simulink model "SystemPartModel"  (Simulink 8.8)
settings: Solver=VariableStepAuto  StartTime=0.0  StopTime=24*6  RelTol=1e-3
libraries: mpclib x1
settings Model: Creator=zhu  LastModifiedBy=山楂
settings SolverCC: ZeroCrossAlgorithm=Adaptive
settings DataIOCC: LimitDataPoints=off  SaveFormat=Dataset  SignalLoggingSaveFormat=Dataset  ReturnWorkspaceOutputs=on
settings OptimizationCC: LifeSpan=auto
settings DebuggingCC: UnderspecifiedInitializationDetection=Simplified  MergeDetectMultiDrivingBlocksExec=error  IgnoredZcDiagnostic=none  FcnCallInpInsideContextMsg=error  StateNameClashWarn=none  SFUnexpectedBacktrackingDiag=error  SFNoUnconditionalDefaultTransitionDiag=error  SFExecutionAtInitializationDiag=warning
settings HardwareCC: ProdBitPerPointer=64  ProdBitPerSizeT=64  ProdBitPerPtrDiffT=64  ProdLargestAtomicFloat=Float  ProdIntDivRoundTo=Zero  ProdEndianess=LittleEndian  ProdWordSize=64  ProdHWDeviceType=Intel->x86-64 (Windows64)
settings ModelReferenceCC: PropagateSignalLabelsOutOfModel=on
settings SFSimCC: SimUseLocalCustomCode=on
settings RTWCC: RTWUseLocalCustomCode=on
settings GRTTargetCC: TargetLangStandard=C99 (ISO)  CombineOutputUpdateFcns=on  GRTInterface=off
settings ConfigComp: CovMetricSettings=dwe  CovSaveCumulativeToWorkspaceVar=off  CovSaveSingleToWorkspaceVar=off  CovExternalEMLEnable=on

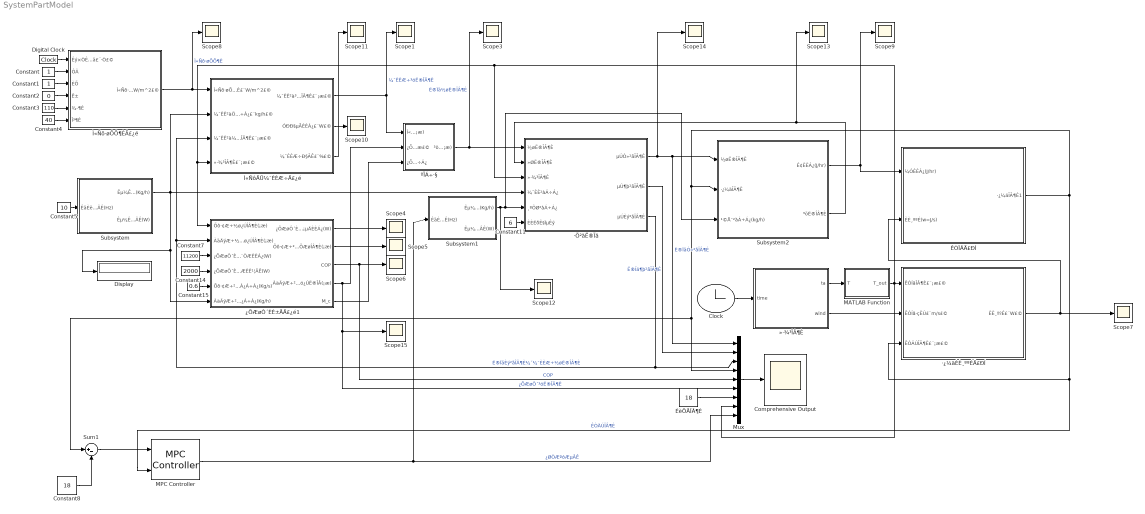
== system SystemPartModel ==
  Clock : Clock
      mask Display: image('$imagefile'); % Use "Edit Image" on toolstrip to change.
  Comprehensive Output : Scope
  Constant : Constant
  Constant1 : Constant
  Constant11 : Constant  Value=6
  Constant14 : Constant  Value=2000
  Constant15 : Constant  Value=0.6
  Constant2 : Constant  Value=0
  Constant3 : Constant  Value=110
  Constant4 : Constant  Value=40
  Constant5 : Constant  Value=10
  Constant7 : Constant  Value=11200
  Constant8 : Constant  Value=18
  Digital Clock : DigitalClock
  Display : Display
  MATLAB Function : MATLAB Function  TreatAsAtomicUnit=on
  MPC Controller : mpclib/MPC Controller  SCDEnableBlockLinearizationSpecification=on  is_multiple=0  enable_value=0  return_u0=off  updateMPCinCallerWorkspace=on  md_inport=off  mv_inport=off  uref_inport=off  cost_outport=off  return_sequence=off  return_qpstatus=off  return_xseq=off  return_state=off  return_ovseq=off  state_inport=off  umin_inport=off  umax_inport=off  ymin_inport=off  ymax_inport=off  cc_inport=off  ywt_inport=off  uwt_inport=off  duwt_inport=off  rhoeps_inport=off  pm_inport=off  MaximumP=10  HorizonChoice=FixedHorizon  n_ts=1  n_p=10  n_mv=1  n_md=1  n_ud=0  n_mo=1  n_uo=0  BlockDataType=double  SampleTimeInherited=off  switch_inport=off
  Mux : Mux  Inputs=9
  Scope{1,3..15} (14 alike) : Scope
  Subsystem : Subsystem
      mask Display: image('$imagefile'); % Use "Edit Image" on toolstrip to change.
  Subsystem1 : Subsystem
      mask Display: image('$imagefile'); % Use "Edit Image" on toolstrip to change.
  Subsystem2 : Subsystem
  Sum1 : Sum  Inputs=|+-
  分层水箱 : Subsystem
      mask Display: image('$imagefile'); % Use "Edit Image" on toolstrip to change.
  合流阀 : Subsystem
      mask Display: image('$imagefile'); % Use "Edit Image" on toolstrip to change.
  太阳能集热器模块 : Subsystem  mask{cw=4187, Ac=40, Mc=1000, UL=1, tau_alpha=0.86}
      mask prompts: cw "水定压比热容，J/kg*℃"; Ac "集热面积，m^2"; Mc "集热器贮水质量，kg"; UL "集热器热损系数，W/m^2"; tau_alpha "透射比和吸收比乘积有效系数"
      mask DialogControl DescGroupVar Prompt: 太阳能集热器模块
      mask Display: image('$imagefile'); % Use "Edit Image" on toolstrip to change.
  太阳辐照度模块 : Subsystem
      mask Display: image('$imagefile'); % Use "Edit Image" on toolstrip to change.
  室温模型 : Subsystem  mask{rou=1.29, ca=1003, V=423}
      mask prompts: rou "空气密度,kg/m^3"; ca "比热容,J/kg*K"; V "室内容积，m^3"
      mask Display: image('$imagefile'); % Use "Edit Image" on toolstrip to change.
  房间热负荷模型 : Subsystem
      mask Display: image('$imagefile'); % Use "Edit Image" on toolstrip to change.
  环境温度 : MATLAB Function  TreatAsAtomicUnit=on
  空气源热泵模块1 : Subsystem
      mask Display: image('$imagefile'); % Use "Edit Image" on toolstrip to change.
  设置温度 : Constant  Value=18
  wires:
  Digital Clock/1 -> 太阳辐照度模块/1(数字时间（分）)
  Constant/1 -> 太阳辐照度模块/2(月)
  Constant1/1 -> 太阳辐照度模块/3(日)
  Constant2/1 -> 太阳辐照度模块/4(时)
  Constant3/1 -> 太阳辐照度模块/5(经度)
  Constant4/1 -> 太阳辐照度模块/6(纬度)
  太阳辐照度模块/1(太阳辐照度（W/m^2）) -> Scope8/1, 太阳能集热器模块/1(太阳辐照度（W/m^2）)  "太阳辐照度"
  合流阀/1(出水温度(℃)) -> 分层水箱/1(进水温度), Scope3/1  "水箱进水温度"
  空气源热泵模块1/5(M_c) -> 合流阀/3(空气源流量)
  空气源热泵模块1/4(冷凝器侧出口水温(℃)) -> Mux/6, Scope15/1, 合流阀/2(空气源侧来水温度(℃）)  "空气源出水温度"
  太阳能集热器模块/1(集热侧出水温度（℃）) -> Scope1/1, 合流阀/1(太阳能侧来水温度(℃))  "集热器出水温度"
  分层水箱/1(第一层温度) -> Scope14/1, Subsystem2/1(进水温度), Mux/1  "水箱一层温度"
  Subsystem2/2(出水温度) -> Scope13/1, 分层水箱/2(回水温度)
  Constant11/1 -> 分层水箱/6(热损失系数)
  Constant7/1 -> 空气源热泵模块1/3(空气源热泵额定制热量(W))
  Constant14/1 -> 空气源热泵模块1/4(空气源热泵额定制热功率(W))
  Constant15/1 -> 空气源热泵模块1/5(蒸发器侧介质的质量流量(Kg/s))
  Mux/1 -> Comprehensive Output/1
  分层水箱/2(第二层温度) -> Mux/2  "水箱二层温度"
  分层水箱/3(第三层温度) -> 空气源热泵模块1/2(冷凝器进口温度(℃)), 太阳能集热器模块/3(集热侧进水温度（℃）), Mux/3  "水箱三层温度即集热器进水温度"
  空气源热泵模块1/1(空气源热泵蒸发器从热源侧提取的热量(W)) -> Scope4/1
  空气源热泵模块1/2(蒸发器侧出口空气温度(℃)) -> Scope5/1
  空气源热泵模块1/3(COP) -> Mux/5, Scope6/1  "COP"
  太阳能集热器模块/2(有效得热量（W）) -> Scope10/1
  太阳能集热器模块/3(集热器效率（%）) -> Scope11/1
  Constant5/1 -> Subsystem/1(输入频率(Hz))
  Subsystem/1(实际输出流量(Kg/h)) -> 太阳能集热器模块/2(集热侧质量流量（kg/h）), 分层水箱/4(集热侧流量), Display/1, 空气源热泵模块1/6(冷凝器侧介质的质量流量(Kg/h))
  环境温度/1(ta) -> MATLAB Function/1(T)
  环境温度/2(wind) -> 房间热负荷模型/2(室外风速（m/s）)
  Clock/1 -> 环境温度/1(time)
  室温模型/1(房间温度1) -> Subsystem2/2(房间温度), Sum1/1, Mux/4, MPC Controller/2, 房间热负荷模型/3(室内温度（℃）)  "室内温度"
  Subsystem1/1(实际输出流量(Kg/h)) -> Scope12/1, Subsystem2/3(供暖侧流量(kg/h)), 分层水箱/5(负载侧流量)
  Subsystem2/1(散热量(J/hr)) -> 室温模型/1(加热量(J/hr)), Scope9/1
  设置温度/1 -> Mux/7
  房间热负荷模型/1(热负荷（W）) -> 室温模型/2(热负荷(w=J/s)), Scope7/1
  MPC Controller/1 -> Mux/9, Subsystem1/1(输入频率(Hz))  "控制后频率"
  Constant8/1 -> Sum1/2
  MATLAB Function/1(T_out) -> Mux/8, 房间热负荷模型/1(室外温度（℃）), 分层水箱/3(环境温度), 空气源热泵模块1/1(蒸发器进口温度(℃)), 太阳能集热器模块/4(环境温度（℃）)
  Sum1/1 -> MPC Controller/1

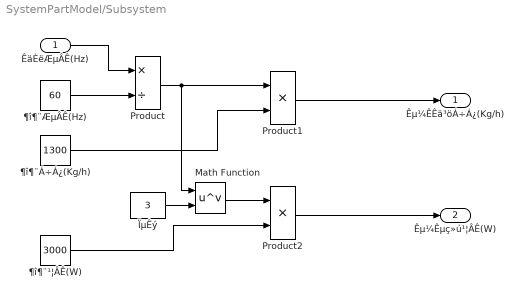
== system SystemPartModel/Subsystem ==
  输入频率(Hz) : Inport
  Math Function : Math  Operator=pow  SaturateOnIntegerOverflow=on
  Product : Product  Inputs=*/
  Product1 : Product
  Product2 : Product
  系数 : Constant  Value=3
  额定功率(W) : Constant  Value=3000
  额定流量(Kg/h) : Constant  Value=1300
  额定频率(Hz) : Constant  Value=60
  实际输出流量(Kg/h) : Outport
  实际电机功率(W) : Outport  Port=2
  wires:
  系数/1 -> Math Function/2
  Math Function/1 -> Product2/1
  额定频率(Hz)/1 -> Product/2
  额定流量(Kg/h)/1 -> Product1/2
  Product/1 -> Math Function/1, Product1/1
  额定功率(W)/1 -> Product2/2
  Product2/1 -> 实际电机功率(W)/1
  输入频率(Hz)/1 -> Product/1
  Product1/1 -> 实际输出流量(Kg/h)/1

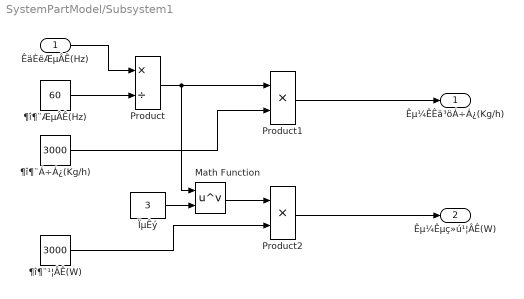
== system SystemPartModel/Subsystem1 ==
  输入频率(Hz) : Inport
  Math Function : Math  Operator=pow  SaturateOnIntegerOverflow=on
  Product : Product  Inputs=*/
  Product1 : Product
  Product2 : Product
  系数 : Constant  Value=3
  额定功率(W) : Constant  Value=3000
  额定流量(Kg/h) : Constant  Value=3000
  额定频率(Hz) : Constant  Value=60
  实际输出流量(Kg/h) : Outport
  实际电机功率(W) : Outport  Port=2
  wires:
  Product1/1 -> 实际输出流量(Kg/h)/1
  输入频率(Hz)/1 -> Product/1
  Product2/1 -> 实际电机功率(W)/1
  额定功率(W)/1 -> Product2/2
  Product/1 -> Product1/1, Math Function/1
  额定流量(Kg/h)/1 -> Product1/2
  额定频率(Hz)/1 -> Product/2
  Math Function/1 -> Product2/1
  系数/1 -> Math Function/2

== system SystemPartModel/Subsystem2 ==
  进水温度 : Inport
  房间温度 : Inport  Port=2
  供暖侧流量(kg/h) : Inport  Port=3
  Constant : Constant  Value=7.77
  Subsystem : Subsystem
  Subsystem1 : Subsystem
  散热量(J/hr) : Outport
  出水温度 : Outport  Port=2
  wires:
  房间温度/1 -> Subsystem/2(房间温度)
  进水温度/1 -> Subsystem1/3(进水温度), Subsystem/1(进水温度)
  Constant/1 -> ?
  Subsystem1/1(出水温度) -> 出水温度/1
  供暖侧流量(kg/h)/1 -> Subsystem1/2(供热流量(kg/h)), Subsystem/3(供热流量，kg/h)
  Subsystem/1(散热量(j/hr)) -> 散热量(J/hr)/1, Subsystem1/1(散热量)

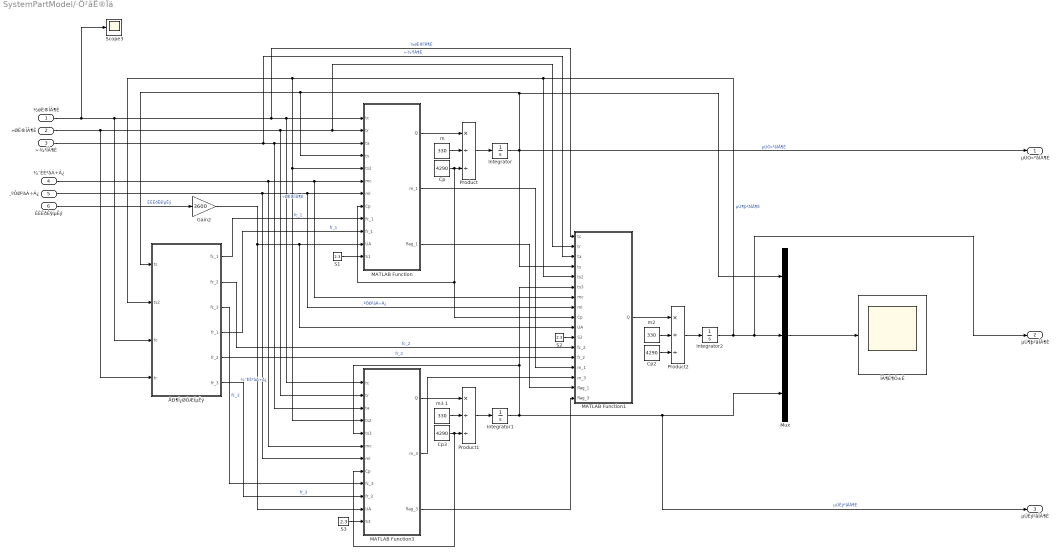
== system SystemPartModel/分层水箱 ==
  进水温度 : Inport
  回水温度 : Inport  Port=2
  环境温度 : Inport  Port=3
  集热侧流量 : Inport  Port=4
  负载侧流量 : Inport  Port=5
  热损失系数 : Inport  Port=6
  Cp : Constant  Value=4290
  Cp2 : Constant  Value=4290
  Cp3 : Constant  Value=4290
  Gain2 : Gain  Gain=3600
  Integrator : Integrator  InitialCondition=45
  Integrator1 : Integrator  InitialCondition=45
  Integrator2 : Integrator  InitialCondition=45
  MATLAB Function : MATLAB Function  TreatAsAtomicUnit=on
  MATLAB Function1 : MATLAB Function  TreatAsAtomicUnit=on
  MATLAB Function3 : MATLAB Function  TreatAsAtomicUnit=on
  Mux : Mux  Inputs=3
  Product : Product  Inputs=*//
  Product1 : Product  Inputs=*//
  Product2 : Product  Inputs=*//
  S1 : Constant  Value=2.3
  S2 : Constant  Value=2.3
  S3 : Constant  Value=2.3
  Scope3 : Scope
  "m " : Constant  Value=330
  m2 : Constant  Value=330
  m3 1 : Constant  Value=330
  判断控制系数 : MATLAB Function  TreatAsAtomicUnit=on
  温度对比 : Scope
  第一层温度 : Outport
  第二层温度 : Outport  Port=2
  第三层温度 : Outport  Port=3
  wires:
  Integrator1/1 -> 第三层温度/1, Mux/3, MATLAB Function1/6(ts3), MATLAB Function3/5(ts3)  "第三层温度"
  Integrator2/1 -> 第二层温度/1, Mux/2, MATLAB Function1/5(ts2), MATLAB Function3/4(ts2), MATLAB Function/5(ts2), 判断控制系数/2(ts2)  "第二层温度"
  Product/1 -> Integrator/1
  负载侧流量/1 -> MATLAB Function3/7(ml), MATLAB Function1/8(ml), MATLAB Function/7(ml)  "负载侧流量"
  Integrator/1 -> 第一层温度/1, MATLAB Function/4(ts), 判断控制系数/1(ts), Mux/1, MATLAB Function1/4(ts)  "第一层温度"
  Mux/1 -> 温度对比/1
  MATLAB Function/3(flag_1) -> MATLAB Function1/16(flag_1)
  "m "/1 -> Product/2
  判断控制系数/5(fr_2) -> MATLAB Function1/13(fr_2)  "fr_2"
  MATLAB Function3/1(Q) -> Product1/1
  判断控制系数/4(fr_1) -> MATLAB Function/10(fr_1)  "fr_1"
  环境温度/1 -> MATLAB Function1/3(ta), MATLAB Function3/3(ta), MATLAB Function/3(ta)  "环境温度"
  判断控制系数/1(fc_1) -> MATLAB Function/9(fc_1)  "fc_1"
  MATLAB Function3/3(flag_3) -> MATLAB Function1/17(flag_3)
  Product1/1 -> Integrator1/1
  判断控制系数/3(fc_3) -> MATLAB Function3/9(fc_3)  "fc_3"
  回水温度/1 -> 判断控制系数/4(tr), MATLAB Function1/2(tr), MATLAB Function/2(tr), MATLAB Function3/2(tr)  "回水温度"
  m3 1/1 -> Product1/2
  MATLAB Function1/1(Q) -> Product2/1
  Cp3/1 -> MATLAB Function3/8(Cp), Product1/3
  MATLAB Function/1(Q) -> Product/1
  判断控制系数/2(fc_2) -> MATLAB Function1/12(fc_2)  "fc_2"
  m2/1 -> Product2/2
  Cp2/1 -> Product2/3
  判断控制系数/6(fr_3) -> MATLAB Function3/10(fr_3)  "fr_3"
  热损失系数/1 -> Gain2/1  "热损失系数"
  Cp/1 -> MATLAB Function1/9(Cp), MATLAB Function/8(Cp), Product/3
  S1/1 -> MATLAB Function/12(S1)
  S3/1 -> MATLAB Function3/12(S3)
  集热侧流量/1 -> MATLAB Function3/6(mc), MATLAB Function1/7(mc), MATLAB Function/6(mc)  "集热侧流量"
  S2/1 -> MATLAB Function1/11(S2)
  MATLAB Function3/2(m_3) -> MATLAB Function1/15(m_3)
  进水温度/1 -> Scope3/1, 判断控制系数/3(tc), MATLAB Function1/1(tc), MATLAB Function3/1(tc), MATLAB Function/1(tc)  "进水温度"
  MATLAB Function/2(m_1) -> MATLAB Function1/14(m_1)
  Product2/1 -> Integrator2/1
  Gain2/1 -> MATLAB Function3/11(UA), MATLAB Function1/10(UA), MATLAB Function/11(UA)

== system SystemPartModel/合流阀 ==
  太阳能侧来水温度(℃) : Inport
  空气源侧来水温度(℃） : Inport  Port=2
  空气源流量 : Inport  Port=3
  MATLAB Function : MATLAB Function  TreatAsAtomicUnit=on
  出水温度(℃) : Outport
  wires:
  太阳能侧来水温度(℃)/1 -> MATLAB Function/1(c_in)
  空气源侧来水温度(℃）/1 -> MATLAB Function/2(a_in)
  MATLAB Function/1(t_out) -> 出水温度(℃)/1
  空气源流量/1 -> MATLAB Function/3(m_c)

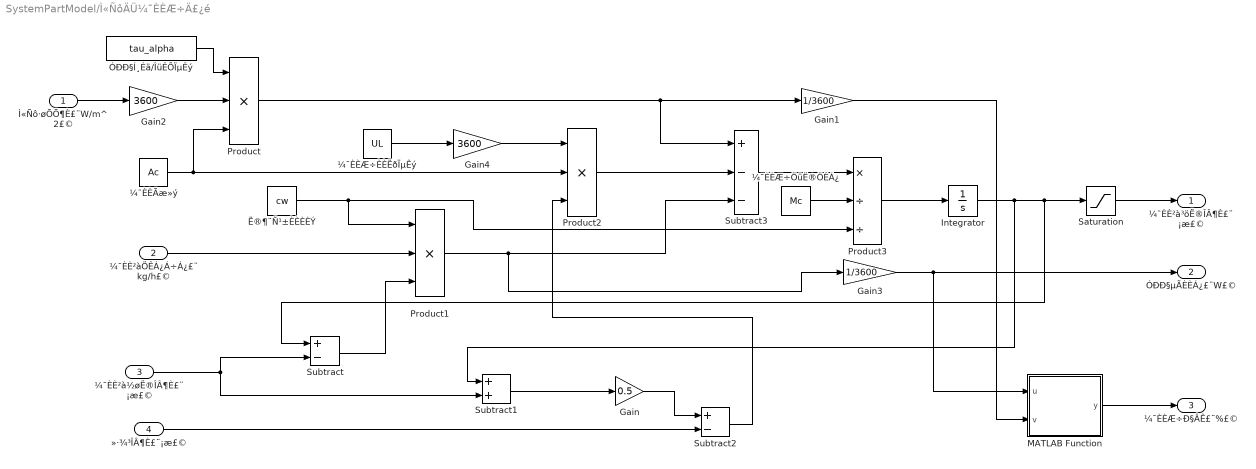
== system SystemPartModel/太阳能集热器模块 ==
  太阳辐照度（W/m^2） : Inport
  集热侧质量流量（kg/h） : Inport  Port=2
  集热侧进水温度（℃） : Inport  Port=3
  环境温度（℃） : Inport  Port=4
  Gain : Gain  Gain=0.5
  Gain1 : Gain  Gain=1/3600
  Gain2 : Gain  Gain=3600
  Gain3 : Gain  Gain=1/3600
  Gain4 : Gain  Gain=3600
  Integrator : Integrator
  MATLAB Function : MATLAB Function  TreatAsAtomicUnit=on
  Product : Product  Inputs=3
  Product1 : Product  Inputs=3
  Product2 : Product  Inputs=3
  Product3 : Product  Inputs=*//
  Saturation : Saturate  UpperLimit=100  LowerLimit=0
  Subtract : Sum  Inputs=+-
  Subtract1 : Sum
  Subtract2 : Sum  Inputs=+-
  Subtract3 : Sum  Inputs=+--
  有效透射/吸收系数 : Constant  Value=tau_alpha
  水定压比热容 : Constant  Value=cw
  集热器热损系数 : Constant  Value=UL
  集热器贮水质量 : Constant  Value=Mc
  集热面积 : Constant  Value=Ac
  集热侧出水温度（℃） : Outport
  有效得热量（W） : Outport  Port=2
  集热器效率（%） : Outport  Port=3
  wires:
  Product1/1 -> Subtract3/3, Gain3/1
  Integrator/1 -> Subtract1/1, Subtract/1, Saturation/1
  有效透射/吸收系数/1 -> Product/1
  Subtract/1 -> Product1/3
  集热器热损系数/1 -> Gain4/1
  Product2/1 -> Subtract3/2
  集热器贮水质量/1 -> Product3/2
  太阳辐照度（W/m^2）/1 -> Gain2/1
  Gain/1 -> Subtract2/1
  Subtract2/1 -> Product2/3
  Product3/1 -> Integrator/1
  Subtract1/1 -> Gain/1
  环境温度（℃）/1 -> Subtract2/2
  Subtract3/1 -> Product3/1
  集热侧进水温度（℃）/1 -> Subtract/2, Subtract1/2
  集热面积/1 -> Product2/2, Product/3
  水定压比热容/1 -> Product1/1, Product3/3
  Gain2/1 -> Product/2
  集热侧质量流量（kg/h）/1 -> Product1/2
  Gain4/1 -> Product2/1
  Gain3/1 -> MATLAB Function/1(u), 有效得热量（W）/1
  Product/1 -> Gain1/1, Subtract3/1
  Gain1/1 -> MATLAB Function/2(v)
  MATLAB Function/1(y) -> 集热器效率（%）/1
  Saturation/1 -> 集热侧出水温度（℃）/1

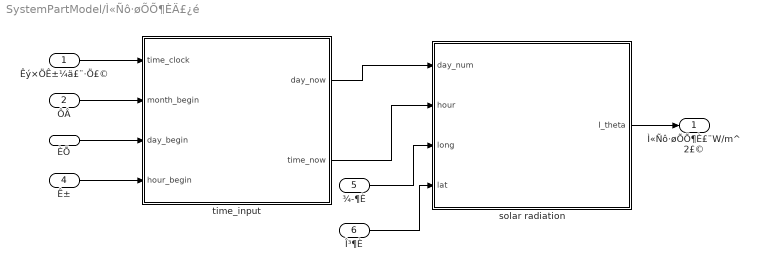
== system SystemPartModel/太阳辐照度模块 ==
  数字时间（分） : Inport
  月 : Inport  Port=2
  日 : Inport  Port=3
  时 : Inport  Port=4
  经度 : Inport  Port=5
  纬度 : Inport  Port=6
  "solar radiation " : MATLAB Function  TreatAsAtomicUnit=on
  time_input : MATLAB Function  TreatAsAtomicUnit=on
  太阳辐照度（W/m^2） : Outport
  wires:
  time_input/2(time_now) -> "solar radiation "/2(hour)
  "solar radiation "/1(I_theta) -> 太阳辐照度（W/m^2）/1
  数字时间（分）/1 -> time_input/1(time_clock)
  时/1 -> time_input/4(hour_begin)
  time_input/1(day_now) -> "solar radiation "/1(day_num)
  月/1 -> time_input/2(month_begin)
  日/1 -> time_input/3(day_begin)
  经度/1 -> "solar radiation "/3(long)
  纬度/1 -> "solar radiation "/4(lat)

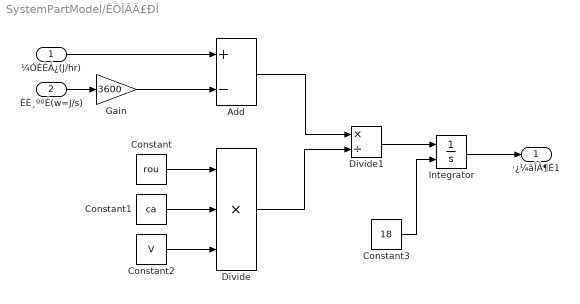
== system SystemPartModel/室温模型 ==
  加热量(J/hr) : Inport
  热负荷(w=J/s) : Inport  Port=2
  Add : Sum  Inputs=+-
  Constant : Constant  Value=rou
  Constant1 : Constant  Value=ca
  Constant2 : Constant  Value=V
  Constant3 : Constant  Value=18
  Divide : Product  Inputs=***
  Divide1 : Product  Inputs=*/
  Gain : Gain  Gain=3600
  Integrator : Integrator  InitialConditionSource=external  InitialCondition=10
  房间温度1 : Outport  OutMax=[25]
  wires:
  Constant2/1 -> Divide/3
  Constant/1 -> Divide/1
  Constant1/1 -> Divide/2
  Divide/1 -> Divide1/2
  加热量(J/hr)/1 -> Add/1
  热负荷(w=J/s)/1 -> Gain/1
  Add/1 -> Divide1/1
  Divide1/1 -> Integrator/1
  Gain/1 -> Add/2
  Constant3/1 -> Integrator/2
  Integrator/1 -> 房间温度1/1

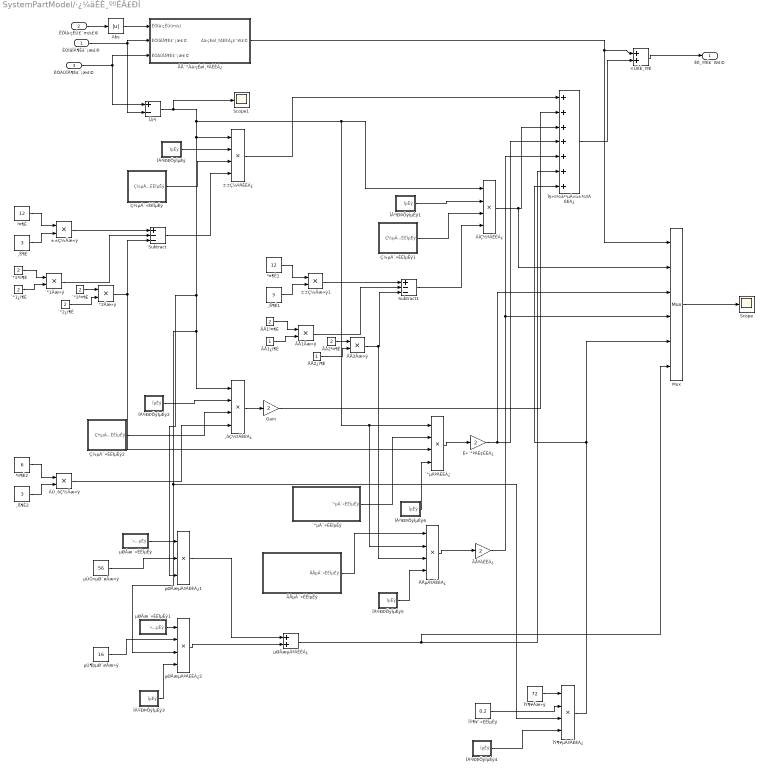
== system SystemPartModel/房间热负荷模型 ==
  室外温度（℃） : Inport
  室外风速（m/s） : Inport  Port=2
  室内温度（℃） : Inport  Port=3
  Abs : Abs
  Gain : Gain  Gain=2
  Mux : Mux  Inputs=6
  Scope : Scope
  Scope1 : Scope
  Subtract : Sum  Inputs=+--
  Subtract1 : Sum  Inputs=+--
  内隔墙面积 : Product
  北墙耗热量 : Product  Inputs=4
  北墙面积 : Product
  北墙面积1 : Product
  南墙耗热量 : Product  Inputs=4
  双窗耗散热量 : Gain  Gain=2
  围护结构的基本耗热量 : Sum  Inputs=7
  地面传热系数 : Subsystem  mask{N=1}
      mask prompts: N "地面计算地带编号，按离外墙的距离，每2m为一个地带。（1~4）"
      mask DialogControl DescTextVar Prompt: 在冬季，室内热量通过靠近外墙地面传到室外的路程较短，热阻较小；而通过远离外墙地面传到室外的路程较长，热阻增大。因此，室内地面的传热系数随着离外墙的远近而有变化，但在离外墙约8m以上的地面，传热量基本不变。
  地面传热系数1 : Subsystem  mask{N=2}
      mask prompts: N "地面计算地带编号，按离外墙的距离，每2m为一个地带。（1~4）"
      mask DialogControl DescTextVar Prompt: 在冬季，室内热量通过靠近外墙地面传到室外的路程较短，热阻较小；而通过远离外墙地面传到室外的路程较长，热阻增大。因此，室内地面的传热系数随着离外墙的远近而有变化，但在离外墙约8m以上的地面，传热量基本不变。
  地面的耗热量 : Sum
  地面的耗热量1 : Product  Inputs=3
  地面的耗热量2 : Product  Inputs=4
  墙的传热系数 : Subsystem  mask{wall_type=1, brick=1}
      mask prompts: wall_type "墙的类型：1外墙；2内墙"; brick "砖的型号：外墙（1 24砖；2 27砖；3 49砖）内墙（1 12砖；2 24砖）"
      mask DialogControl DescGroupVar Prompt: 墙的传热系数
  墙的传热系数1 : Subsystem  mask{wall_type=2, brick=2}
      mask prompts: wall_type "墙的类型：1外墙；2内墙"; brick "砖的型号：外墙（1 24砖；2 27砖；3 49砖）内墙（1 12砖；2 24砖）"
      mask DialogControl DescGroupVar Prompt: 墙的传热系数
  墙的传热系数2 : Subsystem  mask{wall_type=2, brick=2}
      mask prompts: wall_type "墙的类型：1外墙；2内墙"; brick "砖的型号：外墙（1 24砖；2 27砖；3 49砖）内墙（1 12砖；2 24砖）"
      mask DialogControl DescGroupVar Prompt: 墙的传热系数
  屋顶传热系数 : Constant  Value=0.2
  屋顶的耗热量 : Product  Inputs=4
  屋顶面积 : Constant  Value=72
  总热负荷 : Sum
  温差 : Sum  Inputs=+-
  温差修正系数 : Subsystem  mask{alpha=0.5}
      mask prompts: alpha "外墙、屋顶、地面以及与室外相通的楼板等 1.00； 闷顶和室外空气相通的非采暖地下室上面的楼板等 0.90； 非采暖地下室上面的楼板、外墙有窗时 0.75； 非采暖地下窄上面的楼板、外墙无窗且位于室外地坪以上时 0.60； 非采暖地下室上面的楼板、外墙无窗且位于室外地坪以下时 0.40； 与有外门窗的非采暖房间相邻的隔墙 0.70； 与无外门窗的非采暖房间相邻的隔墙 0.40； 伸缩缝墙、沉降缝墙 0.30； 防震缝墙 0.70；"
  温差修正系数1 : Subsystem  mask{alpha=0.7}
      mask prompts: alpha "外墙、屋顶、地面以及与室外相通的楼板等 1.00； 闷顶和室外空气相通的非采暖地下室上面的楼板等 0.90； 非采暖地下室上面的楼板、外墙有窗时 0.75； 非采暖地下窄上面的楼板、外墙无窗且位于室外地坪以上时 0.60； 非采暖地下室上面的楼板、外墙无窗且位于室外地坪以下时 0.40； 与有外门窗的非采暖房间相邻的隔墙 0.70； 与无外门窗的非采暖房间相邻的隔墙 0.40； 伸缩缝墙、沉降缝墙 0.30； 防震缝墙 0.70；"
  温差修正系数2 : Subsystem  mask{alpha=0.2}
      mask prompts: alpha "外墙、屋顶、地面以及与室外相通的楼板等 1.00； 闷顶和室外空气相通的非采暖地下室上面的楼板等 0.90； 非采暖地下室上面的楼板、外墙有窗时 0.75； 非采暖地下窄上面的楼板、外墙无窗且位于室外地坪以上时 0.60； 非采暖地下室上面的楼板、外墙无窗且位于室外地坪以下时 0.40； 与有外门窗的非采暖房间相邻的隔墙 0.70； 与无外门窗的非采暖房间相邻的隔墙 0.40； 伸缩缝墙、沉降缝墙 0.30； 防震缝墙 0.70；"
  温差修正系数3 : Subsystem  mask{alpha=0.4}
      mask prompts: alpha "外墙、屋顶、地面以及与室外相通的楼板等 1.00； 闷顶和室外空气相通的非采暖地下室上面的楼板等 0.90； 非采暖地下室上面的楼板、外墙有窗时 0.75； 非采暖地下窄上面的楼板、外墙无窗且位于室外地坪以上时 0.60； 非采暖地下室上面的楼板、外墙无窗且位于室外地坪以下时 0.40； 与有外门窗的非采暖房间相邻的隔墙 0.70； 与无外门窗的非采暖房间相邻的隔墙 0.40； 伸缩缝墙、沉降缝墙 0.30； 防震缝墙 0.70；"
  温差修正系数4 : Subsystem  mask{alpha=0.4}
      mask prompts: alpha "外墙、屋顶、地面以及与室外相通的楼板等 1.00； 闷顶和室外空气相通的非采暖地下室上面的楼板等 0.90； 非采暖地下室上面的楼板、外墙有窗时 0.75； 非采暖地下窄上面的楼板、外墙无窗且位于室外地坪以上时 0.60； 非采暖地下室上面的楼板、外墙无窗且位于室外地坪以下时 0.40； 与有外门窗的非采暖房间相邻的隔墙 0.70； 与无外门窗的非采暖房间相邻的隔墙 0.40； 伸缩缝墙、沉降缝墙 0.30； 防震缝墙 0.70；"
  温差修正系数5 : Subsystem  mask{alpha=0.6}
      mask prompts: alpha "外墙、屋顶、地面以及与室外相通的楼板等 1.00； 闷顶和室外空气相通的非采暖地下室上面的楼板等 0.90； 非采暖地下室上面的楼板、外墙有窗时 0.75； 非采暖地下窄上面的楼板、外墙无窗且位于室外地坪以上时 0.60； 非采暖地下室上面的楼板、外墙无窗且位于室外地坪以下时 0.40； 与有外门窗的非采暖房间相邻的隔墙 0.70； 与无外门窗的非采暖房间相邻的隔墙 0.40； 伸缩缝墙、沉降缝墙 0.30； 防震缝墙 0.70；"
  温差修正系数6 : Subsystem  mask{alpha=0.6}
      mask prompts: alpha "外墙、屋顶、地面以及与室外相通的楼板等 1.00； 闷顶和室外空气相通的非采暖地下室上面的楼板等 0.90； 非采暖地下室上面的楼板、外墙有窗时 0.75； 非采暖地下窄上面的楼板、外墙无窗且位于室外地坪以上时 0.60； 非采暖地下室上面的楼板、外墙无窗且位于室外地坪以下时 0.40； 与有外门窗的非采暖房间相邻的隔墙 0.70； 与无外门窗的非采暖房间相邻的隔墙 0.40； 伸缩缝墙、沉降缝墙 0.30； 防震缝墙 0.70；"
  窗1宽度 : Constant  Value=2
  窗1长度 : Constant  Value=2
  窗1面积 : Product
  窗2宽度 : Constant  Value=2
  窗2长度 : Constant  Value=2
  窗2面积 : Product
  窗的传热系数 : Subsystem  mask{window_type=2, layers=2}
      mask prompts: window_type "窗的类型：1木框；2金属框；3玻璃窗；4商店橱窗"; layers "层数：1层或2层"
      mask Display: image('C:\Users\Administrator\Desktop\201603301413338053 (1).png'); % Use "Edit Image" on toolstrip to change.
  窗的耗热量 : Product  Inputs=4
  第一地带面积 : Constant  Value=56
  第二地带面积 : Constant  Value=16
  长度 : Constant  Value=12
  长度1 : Constant  Value=12
  长度2 : Constant  Value=6
  门1宽度 : Constant
  门1长度 : Constant  Value=2
  门1面积 : Product
  门2宽度 : Constant
  门2长度 : Constant  Value=2
  门2面积 : Product
  门的传热系数 : Subsystem  mask{door_type=3, layers=1}
      mask prompts: door_type "门的类型：1实体木门；2带玻璃的外门；3内门"; layers "层数：1层或2层"
      mask Display: image('$imagefile'); % Use "Edit Image" on toolstrip to change.
  门的耗热量 : Product  Inputs=4
  门窗冷风渗透耗热量 : Subsystem  mask{Door_type=5, L_door=0.01, city=6, D_door=1, ca=1000}
      mask prompts: Door_type "门窗类型：1单层木；2双层木；3单层钢；4双层钢；5推拉铝；6平开铝"; L_door "门窗缝隙长度（m）"; city "所在城市（就近选择）：1哈尔滨；2沈阳；3北京；4天津；5西安；6太原；7兰州；8乌鲁木齐"; D_door "门窗朝向：1北；2东北；3东；4东南；5南；6 西南； 7西；8 西北"; ca "室外空气定压比热容（J/kg*℃）"
      mask Help: 详情见《供热工程 第四版》第一章，建筑热负荷的计算。
      mask DialogControl DescTextVar Prompt: 在风力和热压造成的室内外压差作用下，室外的冷空气通过们、窗等缝隙渗入室内，被加热后逸出。把这部分冷空气从室外温度加热到室内温度所消耗的热量，称为冷风渗透耗热量。冷风渗透耗热量，在设计热负荷中占有不小的份额。计算冷风渗透耗热量的常用方法有缝隙法、换气法和百分数法，本模块采用缝隙法。
  门耗热量 : Gain  Gain=2
  隔墙耗热量 : Product  Inputs=4
  高度 : Constant  Value=3
  高度1 : Constant  Value=3
  高度2 : Constant  Value=3
  热负荷（W） : Outport
  wires:
  室内温度（℃）/1 -> 温差/1, 门窗冷风渗透耗热量/3(室内温度（℃）)
  室外风速（m/s）/1 -> Abs/1
  室外温度（℃）/1 -> 温差/2, 门窗冷风渗透耗热量/2(室外温度（℃）)
  窗的传热系数/1(窗的传热系数) -> 窗的耗热量/2
  墙的传热系数/1(墙的传热系数) -> 北墙耗热量/3
  长度/1 -> 北墙面积/1
  高度/1 -> 北墙面积/2
  窗1长度/1 -> 窗1面积/1
  窗1宽度/1 -> 窗1面积/2
  窗2长度/1 -> 窗2面积/1
  窗2宽度/1 -> 窗2面积/2
  北墙面积/1 -> Subtract/1
  窗1面积/1 -> Subtract/2
  窗2面积/1 -> Subtract/3, 窗的耗热量/3
  温差修正系数/1(系数) -> 北墙耗热量/2
  Subtract/1 -> 北墙耗热量/4
  门1宽度/1 -> 门1面积/2
  门1面积/1 -> Subtract1/2
  门2长度/1 -> 门2面积/1
  门2宽度/1 -> 门2面积/2
  Subtract1/1 -> 南墙耗热量/4
  北墙面积1/1 -> Subtract1/1
  门2面积/1 -> 门的耗热量/3, Subtract1/3
  长度1/1 -> 北墙面积1/1
  墙的传热系数1/1(墙的传热系数) -> 南墙耗热量/3
  温差修正系数1/1(系数) -> 南墙耗热量/2
  高度1/1 -> 北墙面积1/2
  门1长度/1 -> 门1面积/1
  温差修正系数2/1(系数) -> 隔墙耗热量/2
  墙的传热系数2/1(墙的传热系数) -> 隔墙耗热量/3
  长度2/1 -> 内隔墙面积/1
  高度2/1 -> 内隔墙面积/2
  内隔墙面积/1 -> 隔墙耗热量/4
  隔墙耗热量/1 -> Gain/1
  窗的耗热量/1 -> 双窗耗散热量/1
  门的耗热量/1 -> 门耗热量/1
  门的传热系数/1(门的传热系数) -> 门的耗热量/1
  北墙耗热量/1 -> 围护结构的基本耗热量/1
  Gain/1 -> 围护结构的基本耗热量/2
  南墙耗热量/1 -> Mux/2, 围护结构的基本耗热量/3
  双窗耗散热量/1 -> Mux/3, 围护结构的基本耗热量/4
  门耗热量/1 -> Mux/4, 围护结构的基本耗热量/5
  地面传热系数/1(传热系数) -> 地面的耗热量1/1
  第一地带面积/1 -> 地面的耗热量1/2
  地面传热系数1/1(传热系数) -> 地面的耗热量2/1
  第二地带面积/1 -> 地面的耗热量2/2
  地面的耗热量1/1 -> 地面的耗热量/1
  地面的耗热量2/1 -> 地面的耗热量/2
  地面的耗热量/1 -> Mux/6, 围护结构的基本耗热量/6
  屋顶的耗热量/1 -> Mux/5, 围护结构的基本耗热量/7
  屋顶传热系数/1 -> 屋顶的耗热量/2
  屋顶面积/1 -> 屋顶的耗热量/1
  温差/1 -> Scope1/1, 南墙耗热量/1, 门的耗热量/2, 窗的耗热量/1, 地面的耗热量1/3, 地面的耗热量2/3, 屋顶的耗热量/3, 隔墙耗热量/1, 北墙耗热量/1
  围护结构的基本耗热量/1 -> 总热负荷/2
  门窗冷风渗透耗热量/1(冷风渗透耗热量（W）) -> Mux/1, 总热负荷/1
  总热负荷/1 -> 热负荷（W）/1
  Mux/1 -> Scope/1
  Abs/1 -> 门窗冷风渗透耗热量/1(室外风速(m/s))
  温差修正系数3/1(系数) -> 地面的耗热量2/4
  温差修正系数4/1(系数) -> 屋顶的耗热量/4
  温差修正系数5/1(系数) -> 门的耗热量/4
  温差修正系数6/1(系数) -> 窗的耗热量/4

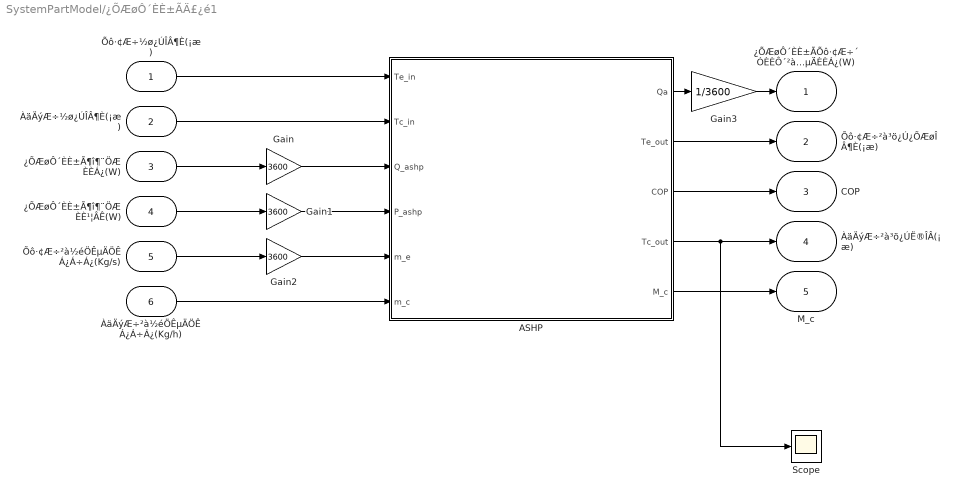
== system SystemPartModel/空气源热泵模块1 ==
  蒸发器进口温度(℃) : Inport
  冷凝器进口温度(℃) : Inport  Port=2
  空气源热泵额定制热量(W) : Inport  Port=3
  空气源热泵额定制热功率(W) : Inport  Port=4
  蒸发器侧介质的质量流量(Kg/s) : Inport  Port=5
  冷凝器侧介质的质量流量(Kg/h) : Inport  Port=6
  ASHP : MATLAB Function  TreatAsAtomicUnit=on
  Gain : Gain  Gain=3600
  Gain1 : Gain  Gain=3600
  Gain2 : Gain  Gain=3600
  Gain3 : Gain  Gain=1/3600
  Scope : Scope
  空气源热泵蒸发器从热源侧提取的热量(W) : Outport
  蒸发器侧出口空气温度(℃) : Outport  Port=2
  COP : Outport  Port=3
  冷凝器侧出口水温(℃) : Outport  Port=4
  M_c : Outport  Port=5
  wires:
  ASHP/2(Te_out) -> 蒸发器侧出口空气温度(℃)/1
  蒸发器侧介质的质量流量(Kg/s)/1 -> Gain2/1
  ASHP/3(COP) -> COP/1
  冷凝器进口温度(℃)/1 -> ASHP/2(Tc_in)
  空气源热泵额定制热功率(W)/1 -> Gain1/1
  ASHP/4(Tc_out) -> Scope/1, 冷凝器侧出口水温(℃)/1
  ASHP/1(Qa) -> Gain3/1
  空气源热泵额定制热量(W)/1 -> Gain/1
  蒸发器进口温度(℃)/1 -> ASHP/1(Te_in)
  Gain/1 -> ASHP/3(Q_ashp)
  Gain1/1 -> ASHP/4(P_ashp)
  Gain2/1 -> ASHP/5(m_e)
  冷凝器侧介质的质量流量(Kg/h)/1 -> ASHP/6(m_c)
  ASHP/5(M_c) -> M_c/1
  Gain3/1 -> 空气源热泵蒸发器从热源侧提取的热量(W)/1

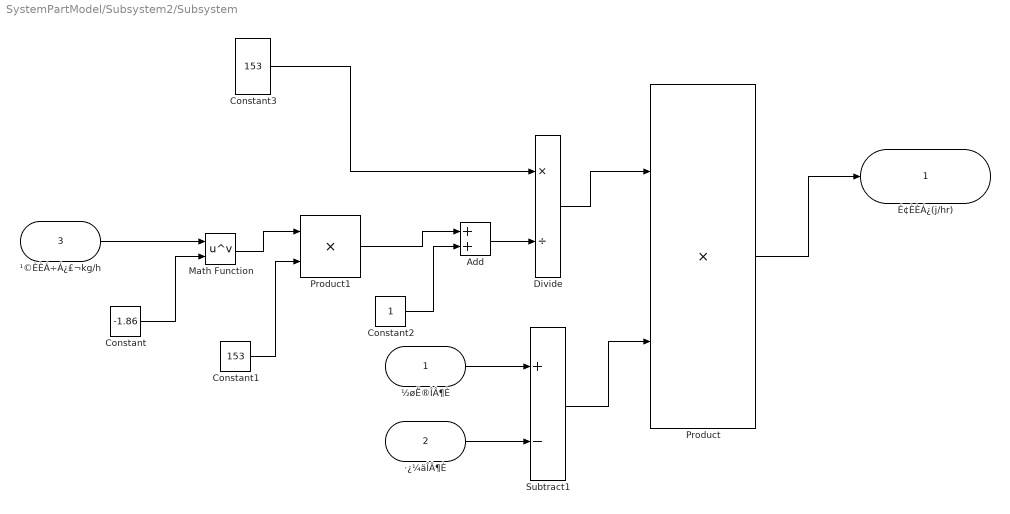
== system SystemPartModel/Subsystem2/Subsystem ==
  进水温度 : Inport
  房间温度 : Inport  Port=2
  供热流量，kg/h : Inport  Port=3
  Add : Sum
  Constant : Constant  Value=-1.86
  Constant1 : Constant  Value=153
  Constant2 : Constant
  Constant3 : Constant  Value=153
  Divide : Product  Inputs=*/
  Math Function : Math  Operator=pow  SaturateOnIntegerOverflow=on
  Product : Product
  Product1 : Product
  Subtract1 : Sum  Inputs=+-
  散热量(j/hr) : Outport
  wires:
  房间温度/1 -> Subtract1/2
  Product/1 -> 散热量(j/hr)/1
  Constant/1 -> Math Function/2
  供热流量，kg/h/1 -> Math Function/1
  进水温度/1 -> Subtract1/1
  Math Function/1 -> Product1/1
  Constant1/1 -> Product1/2
  Product1/1 -> Add/1
  Constant2/1 -> Add/2
  Constant3/1 -> Divide/1
  Add/1 -> Divide/2
  Divide/1 -> Product/1
  Subtract1/1 -> Product/2

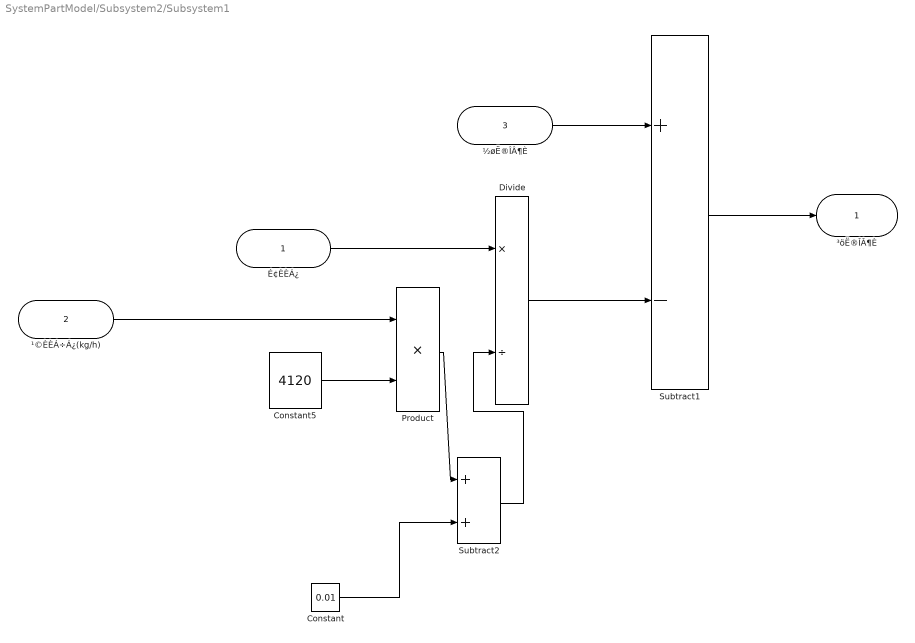
== system SystemPartModel/Subsystem2/Subsystem1 ==
  散热量 : Inport
  供热流量(kg/h) : Inport  Port=2
  进水温度 : Inport  Port=3
  Constant : Constant  Value=0.01
  Constant5 : Constant  Value=4120
  Divide : Product  Inputs=*/
  Product : Product
  Subtract1 : Sum  Inputs=+-
  Subtract2 : Sum
  出水温度 : Outport
  wires:
  Constant5/1 -> Product/2
  Subtract1/1 -> 出水温度/1
  进水温度/1 -> Subtract1/1
  Divide/1 -> Subtract1/2
  散热量/1 -> Divide/1
  Product/1 -> Subtract2/1
  Constant/1 -> Subtract2/2
  Subtract2/1 -> Divide/2
  供热流量(kg/h)/1 -> Product/1

== system SystemPartModel/房间热负荷模型/地面传热系数 ==
  地带区域编号 : Constant  Value=N
  地面的传热系数 : Lookup_n-D  NumberOfTableDimensions=1  BreakpointsForDimension1=[1,2,3,4]  Table=[0.47,0.23,0.12,0.07]  InternalRulePriority=Speed  RndMeth=Simplest  InputSameDT=on
  传热系数 : Outport
  wires:
  地带区域编号/1 -> 地面的传热系数/1
  地面的传热系数/1 -> 传热系数/1

== system SystemPartModel/房间热负荷模型/地面传热系数1 ==
  地带区域编号 : Constant  Value=N
  地面的传热系数 : Lookup_n-D  NumberOfTableDimensions=1  BreakpointsForDimension1=[1,2,3,4]  Table=[0.47,0.23,0.12,0.07]  InternalRulePriority=Speed  RndMeth=Simplest  InputSameDT=on
  传热系数 : Outport
  wires:
  地面的传热系数/1 -> 传热系数/1
  地带区域编号/1 -> 地面的传热系数/1

== system SystemPartModel/房间热负荷模型/墙的传热系数 ==
  墙的传热系数(W/(m^2*℃)) : Lookup_n-D  BreakpointsForDimension1=[1,2,3,4,5,6]  BreakpointsForDimension2=[1,2,3,4,5,6]  Table=reshape([1,0.7,0.6,0.4,0.2,0,2,1.4,1.5,1.1,0.5,0.1,3.1,2.2,2.6,1.8,1,0.3,4.3,3,3.9,2.7,1.6,0.4,5.5,3.9,5.2,3.6,2.3,0.6,6.7,4.7,6.7,4.7,2.9,0.8],6,6)  InternalRulePriority=Speed  RndMeth=Simplest  InputSameDT=on
  墙的类型 : Constant  Value=wall_type
  砖型 : Constant  Value=brick
  墙的传热系数 : Outport
  wires:
  砖型/1 -> 墙的传热系数(W/(m^2*℃))/2
  墙的传热系数(W/(m^2*℃))/1 -> 墙的传热系数/1
  墙的类型/1 -> 墙的传热系数(W/(m^2*℃))/1

== system SystemPartModel/房间热负荷模型/墙的传热系数1 ==
  墙的传热系数(W/(m^2*℃)) : Lookup_n-D  BreakpointsForDimension1=[1,2,3,4,5,6]  BreakpointsForDimension2=[1,2,3,4,5,6]  Table=reshape([1,0.7,0.6,0.4,0.2,0,2,1.4,1.5,1.1,0.5,0.1,3.1,2.2,2.6,1.8,1,0.3,4.3,3,3.9,2.7,1.6,0.4,5.5,3.9,5.2,3.6,2.3,0.6,6.7,4.7,6.7,4.7,2.9,0.8],6,6)  InternalRulePriority=Speed  RndMeth=Simplest  InputSameDT=on
  墙的类型 : Constant  Value=wall_type
  砖型 : Constant  Value=brick
  墙的传热系数 : Outport
  wires:
  砖型/1 -> 墙的传热系数(W/(m^2*℃))/2
  墙的传热系数(W/(m^2*℃))/1 -> 墙的传热系数/1
  墙的类型/1 -> 墙的传热系数(W/(m^2*℃))/1

== system SystemPartModel/房间热负荷模型/墙的传热系数2 ==
  墙的传热系数(W/(m^2*℃)) : Lookup_n-D  BreakpointsForDimension1=[1,2,3,4,5,6]  BreakpointsForDimension2=[1,2,3,4,5,6]  Table=reshape([1,0.7,0.6,0.4,0.2,0,2,1.4,1.5,1.1,0.5,0.1,3.1,2.2,2.6,1.8,1,0.3,4.3,3,3.9,2.7,1.6,0.4,5.5,3.9,5.2,3.6,2.3,0.6,6.7,4.7,6.7,4.7,2.9,0.8],6,6)  InternalRulePriority=Speed  RndMeth=Simplest  InputSameDT=on
  墙的类型 : Constant  Value=wall_type
  砖型 : Constant  Value=brick
  墙的传热系数 : Outport
  wires:
  砖型/1 -> 墙的传热系数(W/(m^2*℃))/2
  墙的传热系数(W/(m^2*℃))/1 -> 墙的传热系数/1
  墙的类型/1 -> 墙的传热系数(W/(m^2*℃))/1

== system SystemPartModel/房间热负荷模型/温差修正系数 ==
  温差修正 : Constant  Value=alpha
  系数 : Outport
  wires:
  温差修正/1 -> 系数/1

== system SystemPartModel/房间热负荷模型/温差修正系数1 ==
  温差修正 : Constant  Value=alpha
  系数 : Outport
  wires:
  温差修正/1 -> 系数/1

== system SystemPartModel/房间热负荷模型/温差修正系数2 ==
  温差修正 : Constant  Value=alpha
  系数 : Outport
  wires:
  温差修正/1 -> 系数/1

== system SystemPartModel/房间热负荷模型/温差修正系数3 ==
  温差修正 : Constant  Value=alpha
  系数 : Outport
  wires:
  温差修正/1 -> 系数/1

== system SystemPartModel/房间热负荷模型/温差修正系数4 ==
  温差修正 : Constant  Value=alpha
  系数 : Outport
  wires:
  温差修正/1 -> 系数/1

== system SystemPartModel/房间热负荷模型/温差修正系数5 ==
  温差修正 : Constant  Value=alpha
  系数 : Outport
  wires:
  温差修正/1 -> 系数/1

== system SystemPartModel/房间热负荷模型/温差修正系数6 ==
  温差修正 : Constant  Value=alpha
  系数 : Outport
  wires:
  温差修正/1 -> 系数/1

== system SystemPartModel/房间热负荷模型/窗的传热系数 ==
  层数1 : Constant  Value=layers
  窗的传热系数(W/(m^2*℃)) : Lookup_n-D  BreakpointsForDimension1=[1,2,3,4,5,6]  BreakpointsForDimension2=[1,2,3,4,5,6]  Table=reshape([1,0.7,0.6,0.4,0.2,0,2,1.4,1.5,1.1,0.5,0.1,3.1,2.2,2.6,1.8,1,0.3,4.3,3,3.9,2.7,1.6,0.4,5.5,3.9,5.2,3.6,2.3,0.6,6.7,4.7,6.7,4.7,2.9,0.8],6,6)  InternalRulePriority=Speed  RndMeth=Simplest  InputSameDT=on
  窗的类型 : Constant  Value=window_type
  窗的传热系数 : Outport
  wires:
  层数1/1 -> 窗的传热系数(W/(m^2*℃))/2
  窗的类型/1 -> 窗的传热系数(W/(m^2*℃))/1
  窗的传热系数(W/(m^2*℃))/1 -> 窗的传热系数/1

== system SystemPartModel/房间热负荷模型/门的传热系数 ==
  层数 : Constant  Value=layers
  门的传热系数(W/(m^2*℃)) : Lookup_n-D  BreakpointsForDimension1=[1,2,3,4]  BreakpointsForDimension2=[1,2]  Table=reshape([5.82,6.4,3.49,4.65,2.68,3.26,3.49,4.65],4,2)  InternalRulePriority=Speed  RndMeth=Simplest  InputSameDT=on
  门的类型 : Constant  Value=door_type
  门的传热系数 : Outport
  wires:
  门的类型/1 -> 门的传热系数(W/(m^2*℃))/1
  层数/1 -> 门的传热系数(W/(m^2*℃))/2
  门的传热系数(W/(m^2*℃))/1 -> 门的传热系数/1

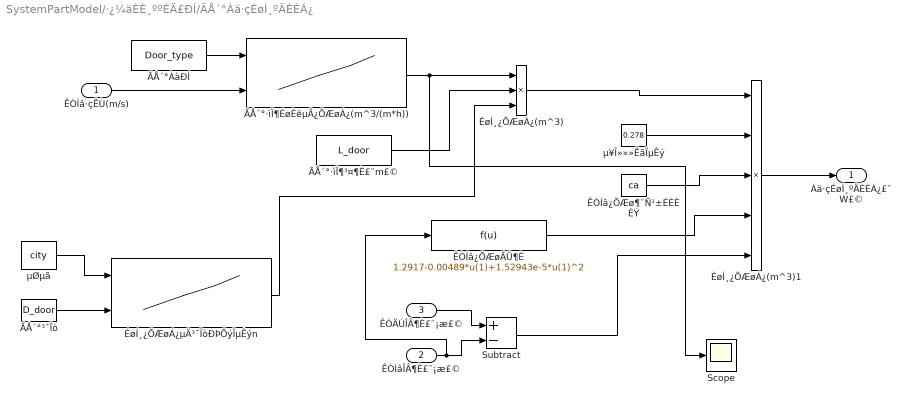
== system SystemPartModel/房间热负荷模型/门窗冷风渗透耗热量 ==
  室外风速(m/s) : Inport
  室外温度（℃） : Inport  Port=2
  室内温度（℃） : Inport  Port=3
  Scope : Scope
  Subtract : Sum  Inputs=+-
  单位换算系数 : Constant  Value=0.278
  地点 : Constant  Value=city
  室外空气定压比热容 : Constant  Value=ca
  室外空气密度 : Fcn  Expr=1.2917-0.00489*u(1)+1.52943e-5*u(1)^2
  渗透空气量(m^3) : Product  Inputs=3
  渗透空气量(m^3)1 : Product  Inputs=5
  渗透空气量的朝向修正系数n : Lookup_n-D  BreakpointsForDimension1=[1,2,3,4,5,6,7,8]  BreakpointsForDimension2=[1,2,3,4,5,6,7,8]  Table=reshape([0.3,1,1,1,0.7,0.9,0.35,0,0.15,0.7,0.5,0.4,1,0.4,1,0.35,0.2,0.3,0.15,0.2,0.7,0.15,1,0.55,0.7,0.3,0.15,0.2,0.7,0.15,1,0.55,1,0.4,0.15,0.15,0.4,0.3,0.5,1,0.85,0.35,0.15,0.2,0.5,0.2,0.2,0.7,0.7,0.3,0.4,0.4,0.35,0.7,0.15,0.25,0.6,0.7,1,1,0.25,1,0.5,0.35],8,8)  InternalRulePriority=Speed  RndMeth=Simplest  InputSameDT=on
  门窗朝向 : Constant  Value=D_door
  门窗类型 : Constant  Value=Door_type
  门窗缝隙渗入的空气量(m^3/(m*h)) : Lookup_n-D  BreakpointsForDimension1=[1,2,3,4,5,6]  BreakpointsForDimension2=[1,2,3,4,5,6]  IndexSearchMethod=Linear search  Table=reshape([1,0.7,0.6,0.4,0.2,0,2,1.4,1.5,1.1,0.5,0.1,3.1,2.2,2.6,1.8,1,0.3,4.3,3,3.9,2.7,1.6,0.4,5.5,3.9,5.2,3.6,2.3,0.6,6.7,4.7,6.7,4.7,2.9,0.8],6,6)  InternalRulePriority=Speed  RndMeth=Simplest  InputSameDT=on
  门窗缝隙长度（m） : Constant  Value=L_door
  冷风渗透耗热量（W） : Outport
  wires:
  门窗类型/1 -> 门窗缝隙渗入的空气量(m^3/(m*h))/1
  单位换算系数/1 -> 渗透空气量(m^3)1/2
  Subtract/1 -> 渗透空气量(m^3)1/5
  门窗朝向/1 -> 渗透空气量的朝向修正系数n/2
  室外风速(m/s)/1 -> 门窗缝隙渗入的空气量(m^3/(m*h))/2
  门窗缝隙长度（m）/1 -> 渗透空气量(m^3)/2
  渗透空气量(m^3)1/1 -> 冷风渗透耗热量（W）/1
  室外空气定压比热容/1 -> 渗透空气量(m^3)1/3
  室内温度（℃）/1 -> Subtract/1
  室外空气密度/1 -> 渗透空气量(m^3)1/4
  地点/1 -> 渗透空气量的朝向修正系数n/1
  渗透空气量的朝向修正系数n/1 -> 渗透空气量(m^3)/3
  室外温度（℃）/1 -> 室外空气密度/1, Subtract/2
  渗透空气量(m^3)/1 -> 渗透空气量(m^3)1/1
  门窗缝隙渗入的空气量(m^3/(m*h))/1 -> Scope/1, 渗透空气量(m^3)/1

== matlab function 太阳辐照度模块/time_input ==
  data: day_now output double; time_clock input double; time_now output double; month_begin input double; day_begin input double; hour_begin input double
%地理位置和时间设置%
%by ShockPig 2021.9.7
%imust

function [day_now,time_now]=initial(time_clock,month_begin,day_begin,hour_begin)

time_all =  time_clock(end);                         %%  运行总小时数

day_all = fix(time_all/24);                          %%  运行总天数
                      
hour_now = rem(hour_begin + rem(time_all,24),24);    %%  rem：除后取余

time_now = hour_now;                                 %%  输出当前时间

day_now  = (month_begin - 1)*30 + day_begin + fix((time_all + hour_begin)/24);     %%  输出当前天数 fix：取整

== matlab function 太阳辐照度模块/solar radiation  ==
  data: day_num input double; hour input double; I_theta output double; long input double; lat input double
%太阳辐照度数学模型%
%by sunguoxin 2020.6.30
%imust

function I_theta =solar_radiation (day_num,hour,long,lat)
 
%%
delta = 23.45*sin((284 + day_num)*360/365); %太阳赤纬角,  deg
delta = delta/57.3; %rad
%%
N0 = 79.6764+ 0.2422*(2020-1985) - fix(2020 - 1985)/4;
theta =  2*pi*(day_num - N0)/365.2422;%日角 rad
E = 0.0028 - 1.9857*sin(theta) + 9.9059*sin(2*theta) - 7.0924*cos(theta) - 0.6882*cos(2*theta); %时差,min
%%
tau_e = hour  -  fix( (120 - long)/15) + fix(E/60);%真太阳时,h
%%
%% 
omiga = (tau_e -12)*15;  %太阳时角,deg
omiga = omiga/57.3; %rad
%% 
phi = lat/57.3;
delta = delta/57.3;
temp = sin(phi)*sin(delta) + cos(phi)*cos(delta)*cos(omiga);
alpha = asin(temp)*57.3; %太阳高度角,deg
alpha = alpha/57.3;%rad
%%
temp = cos(delta)*sin(omiga)/cos(alpha);
if temp >1
    temp = (sin(alpha)*sin(phi) - sin(delta))/(cos(alpha)*cos(phi));
end
gama = acos(temp)*57.3;%太阳方位角,deg
gama = gama/57.3;%rad
%%
theta =20; %斜面与水平面的夹角，默认方位角为0
temp = cos(phi - theta)*cos(delta)*cos(omiga) + sin(phi - theta)*sin(delta);
theta_T = acos(temp)*57.3; %在方位角为0时的太阳入射角,deg
theta_T=theta_T/57.3;%rad
%%
m = 1/sin(alpha);%大气质量
I0 = 1100;%太阳常数,W/m^2
P = 0.8;%大气透明系数
In = I0 * P^m;%$法向直射辐照度,W/m^2
Ib = In*sin(alpha);%水平面直射辐射强度,W/m^2
Ib_T = In*cos(theta_T);%倾斜面直射辐射强度,W/m^2
Id = 0.5*I0*sin(alpha)*(1 - P^m)/(1 - 1.4*log(P)); %水平面散射辐射强度,W/m^2
Id_T = Id*(1 + cos(theta))/2; %倾斜面上散射辐照度，W/m^2
rou = 0.2; %地面反射率
Ir_T = rou*(Ib + Id)*(1- cos(theta))/2;%地面反射辐照度，W/m^2
I_theta = Ib_T + Id_T + Ir_T;%倾斜面上太阳总辐照度
%%
temp = -tan(phi)*sin(delta);
omiga0 = acos(temp)*57.3;
T0 = 12 - fix(omiga0/15);%日出时间
T1 = 12  + fix(omiga0/15);%日落时间
if hour<= T0
    I_theta = 0;
else
    if hour>T1
        I_theta = 0;    
end
end

%%

== matlab function MATLAB Function ==
  data: T input double; T_out output double
function T_out = input(T)


  T_out = T - 5;

== matlab function 太阳能集热器模块/MATLAB Function ==
  data: u input double; y output double; v input double
function y = fcn(u,v)
if v <= 5000
y = 0;
else
   y = u/v;
end

== matlab function 分层水箱/MATLAB Function ==
  data: tc input double; Q output double; tr input double; ta input double; ts input double; ts2 input double; mc input double; ml input double; Cp input double; fc_1 input double; fr_1 input double; UA input double; m_1 output double; flag_1 output double; S1 input double
function [Q,m_1,flag_1]  = first_storey(tc,tr,ta,ts,ts2,mc,ml,Cp,fc_1,fr_1,UA,S1)

m_1 = ml - mc*fc_1 - ml*fr_1;

if m_1>0
    flag_1 = 0;%第2层向第1层供水
else
    flag_1 = 1;%第1层向第2层供水
end

m_1 = abs(m_1);

Q1 = mc * fc_1 * Cp * (tc - ts);%集热侧进水热量
Q2 = (1-flag_1) * m_1 * Cp * (ts2 - ts);%交换水热量
Q3 = ml*fr_1 * Cp * (tr - ts);%用户侧回水热量
Q4 = UA * S1 * (ta-ts);

Q = Q1 + Q2 +Q3 + Q4;%热量变化

== matlab function 分层水箱/MATLAB Function1 ==
  data: tc input double; Q output double; tr input double; ta input double; ts input double; ts2 input double; ts3 input double; mc input double; ml input double; Cp input double; UA input double; S2 input double; fc_2 input double; fr_2 input double; m_1 input double; m_3 input double; flag_1 input double; flag_3 input double
function Q  = second_storey(tc,tr,ta,ts,ts2,ts3,mc,ml,Cp,UA,S2,fc_2,fr_2,m_1,m_3,flag_1,flag_3)

ma = m_1*flag_1;
mb = m_3*flag_3;

Q1 = mc * fc_2 *  Cp * (tc - ts2);%集热侧进水热量
Q2 = ma * Cp * (ts - ts2);%交换水热量1
Q3 = mb * Cp * (ts3 - ts2);%交换水热量2
Q4 = ml * fr_2 * Cp * (tr - ts2);%用户侧回水热量
Q5 = UA * S2 * (ta-ts2);

Q = Q1 + Q2 +Q3 + Q4 +Q5;%水的交换热

== matlab function 分层水箱/MATLAB Function3 ==
  data: tc input double; tr input double; ta input double; ts2 input double; ts3 input double; mc input double; ml input double; Cp input double; fc_3 input double; fr_3 input double; UA input double; Q output double; m_3 output double; flag_3 output double; S3 input double
function [Q,m_3,flag_3]  = third_storey(tc,tr,ta,ts2,ts3,mc,ml,Cp,fc_3,fr_3,UA,S3)

m_3 = mc - mc*fc_3 - ml*fr_3;

if m_3 > 0 
      flag_3 = 0;%第2层向第3层供水
else 
      flag_3 = 1;%第3层向第2层供水
end

m_3 = abs(m_3);

Q1 = mc * fc_3*Cp * (tc - ts3);%集热侧进水热量
Q2 = (1-flag_3) * m_3 * Cp * (ts2 - ts3);%交换水热量
Q3 = ml * fr_3 * Cp * (tr - ts3);%用户侧回水热量
Q4 = UA * S3 * (ta-ts3);

Q = Q1 + Q2 +Q3 + Q4;%水的交换热

== matlab function 分层水箱/判断控制系数 ==
  data: ts input double; ts2 input double; tc input double; fc_1 output double; tr input double; fc_2 output double; fc_3 output double; fr_1 output double; fr_2 output double; fr_3 output double
function [fc_1,fc_2,fc_3,fr_1,fr_2,fr_3] = T(ts,ts2,tc,tr)
    if tc >= ts  %进水口在顶层
        fc_1 = 1;fc_2 = 0;fc_3 = 0;
    else
        if  tc < ts  && tc>=ts2 %进水口在二层
            fc_1 = 0; fc_2 = 1; fc_3 = 0;
         else
            fc_1 = 0;fc_2 = 0;fc_3 = 1;
        end
    end


if tr >= ts  %进水口在顶层
        fr_1 = 1;fr_2 = 0;fr_3 = 0;
    else
        if  tr < ts  && tr>=ts2 %进水口在二层
        fr_1 = 0;fr_2 = 1;fr_3 = 0;
        else
        fr_1 = 0;fr_2 = 0;fr_3 = 1;    
        end
end

== matlab function 空气源热泵模块1/ASHP ==
  data: Te_in input double; Qa output double; Tc_in input double; Q_ashp input double; P_ashp input double; m_e input double; m_c input double; Te_out output double; COP output double; Tc_out output double; M_c output double
function [Qa,Te_out,COP,Tc_out,M_c] = ASHP_input(Te_in,Tc_in,Q_ashp,P_ashp,m_e,m_c)

c_air = 1003;
c_w = 4190;

Qa = Q_ashp - P_ashp;

%COP = Q_ashp / (P_ashp + 0.1);
COP = 1.189*10^(-4)*Te_in^2+0.054*Te_in+3.41;


if Tc_in > 60
    m_e = 0; m_c = 0; Qa = 0; COP = 0;
end


Te_out = Te_in - Qa / (c_air * m_e);

Tc_out = Tc_in + Q_ashp / (c_w * m_c);

if Tc_out > 100
    Tc_out = 100;
end

M_c = m_e;

== matlab function 合流阀/MATLAB Function ==
  data: c_in input double; t_out output double; a_in input double; m_c input double
function t_out  = input(c_in,a_in,m_c)

if m_c == 0
    t_out = c_in;
else
    t_out = (c_in + a_in) / 2;
end

== matlab function 环境温度 ==
  data: ta output double; time input double; wind output double
function [ta,wind] = environment_data(time)

coder.extrinsic('mapminmax');
temp1 = load('environment_data.mat');
temp2 =temp1.environment_data(1:168,:);
X = (1:168);
time_now = 1 + time; 
ta = interp1(X,temp2(1:168,1)',time_now,'linear');
wind = interp1(X,temp2(1:168,3)',time_now,'linear')/10.0;
